simulink model "vendingmachine"  (R2020a)
settings: Solver=FixedStepDiscrete  StartTime=0.0  StopTime=200  FixedStep=0.1  RelTol=1e-3
settings Model: Creator=USER  LastModifiedBy=USER

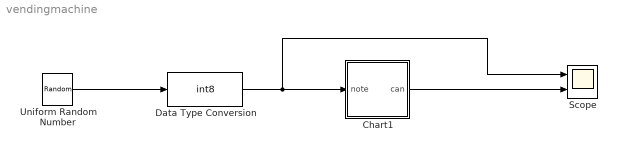
== system vendingmachine ==
  Chart1 : Stateflow chart  TreatAsAtomicUnit=on
  Data Type Conversion : DataTypeConversion  OutDataTypeStr=int8  RndMeth=Nearest  SaturateOnIntegerOverflow=on
  Scope : Scope  NumInputPorts=2
  Uniform Random Number : UniformRandomNumber  Minimum=0  Maximum=2  SampleTime=10
  wires:
  Uniform Random Number/1 -> Data Type Conversion/1
  Data Type Conversion/1 -> Scope/1, Chart1/1(note)
  Chart1/1(can) -> Scope/2

== stateflow chart vendingmachine/Chart1 ==
  settings: stateMachineType=MEALY_MACHINE
  state rupee_zero
  state rupee_Five
  state rupee_Ten
  (default) -> rupee_zero
  rupee_zero -> rupee_Five [order 1] : [note==1]{can=0}
  rupee_Five -> rupee_zero [order 1] : [note==2]{can=1}
  rupee_Ten -> rupee_zero [order 1] : [note==1]{can=1}
  rupee_zero -> rupee_Ten [order 2] : [note==2]{can=0}
  rupee_Ten -> rupee_Five [order 2] : [note==2]{can=1}
  rupee_Five -> rupee_Ten [order 2] : [note==1]{can=0}
  data: can output; note input
